simulink model "autosar_tpc_throttle_sensor2"  (R2022a)
settings: Solver=FixedStepDiscrete  StartTime=0.0  StopTime=10.0  FixedStep=0.005  RelTol=1e-3
model workspace (MATLAB code in the model file + MAT data in the model file):
  TPSPercent_LkupTbl = Simulink.LookupTable
  TPSPercent_LkupTbl.Table.DataType = 'single'
  TPSPercent_LkupTbl.Table.Min = []
  TPSPercent_LkupTbl.Table.Max = []
  TPSPercent_LkupTbl.Table.Unit = ''
  TPSPercent_LkupTbl.Table.FieldName = 'Table'
  TPSPercent_LkupTbl.Table.Description = ''
  TPSPercent_LkupTbl.Table.Value = [0 10 20 30 40 50 60 70 80 90 100]
  TPSPercent_LkupTbl.BreakpointsSpecification = 'Explicit values'
  TPSPercent_LkupTbl.SupportTunableSize = false
  TPSPercent_LkupTbl.Breakpoints.DataType = 'single'
  TPSPercent_LkupTbl.Breakpoints.Min = []
  TPSPercent_LkupTbl.Breakpoints.Max = []
  TPSPercent_LkupTbl.Breakpoints.Unit = ''
  TPSPercent_LkupTbl.Breakpoints.FieldName = 'BP1'
  TPSPercent_LkupTbl.Breakpoints.Description = ''
  TPSPercent_LkupTbl.Breakpoints.Value = single(linspace(170, 966, 11))
  TPSPercent_LkupTbl.Breakpoints.TunableSizeName = 'N1'
  TPSPercent_LkupTbl.CoderInfo.StorageClass = 'Auto'
  TPSPercent_LkupTbl.StructTypeInfo.Name = 'MyStruct'
  TPSPercent_LkupTbl.StructTypeInfo.DataScope = 'Auto'
  TPSPercent_LkupTbl.StructTypeInfo.HeaderFileName = ''
  TPSSecondaryPercent_LkupTbl = Simulink.LookupTable
  TPSSecondaryPercent_LkupTbl.Table = Simulink.lookuptable.Table
  TPSSecondaryPercent_LkupTbl.Table.Value = [100 90 80 70 60 50 40 30 20 10 0]
  TPSSecondaryPercent_LkupTbl.Table.Dimensions = [1 11]
  TPSSecondaryPercent_LkupTbl.Table.DataType = 'single'
  TPSSecondaryPercent_LkupTbl.Table.FieldName = 'Table'
  TPSSecondaryPercent_LkupTbl.Breakpoints = Simulink.lookuptable.Breakpoint
  TPSSecondaryPercent_LkupTbl.Breakpoints.Value = [170 249.600006104 329.200012207 408.799987793 488.399993896 568 647.599975586 727.200012207 806.799987793 886.400024414 966]
  TPSSecondaryPercent_LkupTbl.Breakpoints.TunableSizeName = 'N1'
  TPSSecondaryPercent_LkupTbl.Breakpoints.Dimensions = [1 11]
  TPSSecondaryPercent_LkupTbl.Breakpoints.DataType = 'single'
  TPSSecondaryPercent_LkupTbl.Breakpoints.FieldName = 'BP1'
  TPSSecondaryPercent_LkupTbl.SupportTunableSize = 0
  TPSSecondaryPercent_LkupTbl.StructTypeInfo = Simulink.lookuptable.StructTypeInfo
  TPSSecondaryPercent_LkupTbl.StructTypeInfo.Name = 'MyStruct'
  TPSSecondaryPercent_LkupTbl.StructTypeInfo.DataScope = 'Auto'
  TPSSecondaryPercent_LkupTbl.StructTypeInfo.HeaderFileName = 'Rte_Type.h'
undefined symbols (not defined in the file or in its folder): Dem_EventStatusType, TPSPercentBkpt, TPSPercentTbl
libraries: autosarlibdem x2, autosarlibnvm x1
settings Model: Creator=The MathWorks, Inc.  LastModifiedBy=tsen
settings SolverCC: AlgebraicLoopSolver=TrustRegion
settings DataIOCC: ReturnWorkspaceOutputs=off
settings OptimizationCC: DefaultParameterBehavior=Inlined  PassReuseOutputArgsAs=Individual arguments  ZeroExternalMemoryAtStartup=off  ZeroInternalMemoryAtStartup=off  EfficientTunableParamExpr=on
settings DebuggingCC: ParameterTunabilityLossMsg=error  UnconnectedInputMsg=warning  UnconnectedOutputMsg=warning  UnconnectedLineMsg=warning  SFMachineParentedDataDiag=warning  ArithmeticOperatorsInVariantConditions=warning
settings SFSimCC: SimUseLocalCustomCode=off  MATLABDynamicMemAlloc=off
settings RTWCC: Description=AUTOSAR  SystemTargetFile=autosar.tlc  GenCodeOnly=on  TemplateMakefile=ert_default_tmf  GenerateReport=on  RTWVerbose=off  RTWUseLocalCustomCode=off  IncludeHyperlinkInReport=on  LaunchReport=on  GenerateTraceInfo=on  GenerateTraceReport=on  GenerateTraceReportSl=on  GenerateTraceReportSf=on  GenerateTraceReportEml=on
settings CodeAppCC: ForceParamTrailComments=on  IgnoreCustomStorageClasses=off  OperatorAnnotations=on  SimulinkDataObjDesc=on  SFDataObjDesc=on  InsertBlockDesc=on
settings STFCustomTargetCC: TargetLangStandard=C99 (ISO)  MultiwordLength=256  ParMdlRefBuildCompliant=on  CompOptLevelCompliant=on  IncludeMdlTerminateFcn=off  CombineOutputUpdateFcns=on  SuppressErrorStatus=on  ERTCustomFileBanners=on  SupportNonFinite=off  SupportComplex=off  SupportContinuousTime=off  SupportNonInlinedSFcns=off  RemoveResetFunc=on  MATLABClassNameForMDSCustomization=Simulink.SoftwareTarget.ERTCustomization  CPPClassGenCompliant=on  AutosarCompliant=on  GRTInterface=off  UseToolchainInfoCompliant=on  LookupTableObjectStructAxisOrder=2,1,3,4,...  LUTObjectStructOrderEvenSpacing=Size,Table,Breakpoints  SystemTargetFile=autosar.tlc
settings ERTTargetCC: TargetLangStandard=C99 (ISO)  ConcurrentExecutionCompliant=off  IncludeMdlTerminateFcn=off  SuppressErrorStatus=on  SupportNonFinite=off  SupportComplex=off  ModelStepFunctionPrototypeControlCompliant=off  AutosarCompliant=on  LookupTableObjectStructAxisOrder=2,1,3,4,...  LUTObjectStructOrderEvenSpacing=Size,Table,Breakpoints  InlinedParameterPlacement=NonHierarchical  ERTCustomFileTemplate=example_file_process.tlc

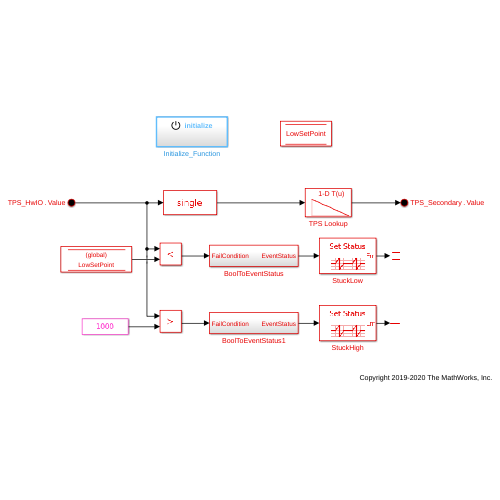
[thumbnail: Simulink's stored preview of the top-level diagram]
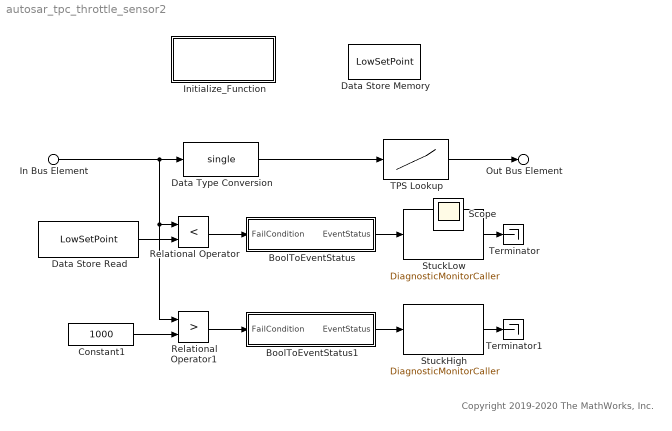
== system autosar_tpc_throttle_sensor2 ==
  note: Copyright 2019-2020 The MathWorks, Inc.
  In Bus Element : Inport  PortName=TPS_HwIO  Element=Value
  BoolToEventStatus : Subsystem
  BoolToEventStatus1 : Subsystem
  Constant1 : Constant  Value=1000
  Data Store Memory : DataStoreMemory  DataStoreName=LowSetPoint  InitialValue=50  ShowAdditionalParam=off
  Data Store Read : DataStoreRead  DataStoreName=LowSetPoint  IndexOptions=Index vector (dialog)  Indices=1  OutputSizes=1
  Data Type Conversion : DataTypeConversion  OutDataTypeStr=single  SaturateOnIntegerOverflow=off  RndMeth=Floor
  Initialize_Function : Subsystem  TreatAsAtomicUnit=on
  Relational Operator : RelationalOperator  Operator=<  OutDataTypeStr=boolean  InputSameDT=off
  Relational Operator1 : RelationalOperator  Operator=>  OutDataTypeStr=boolean  InputSameDT=off
  StuckHigh : autosarlibdem/DiagnosticMonitorCaller  PortName=S2StuckHigh  Operation=SetEventStatus  Datatype=Enum: Dem_EventStatusType  st=-1  ServiceImpl=autosar.bsw.DemDiagnosticMonitor
      settings: SourceProductBaseCode=AS
  StuckLow : autosarlibdem/DiagnosticMonitorCaller  PortName=S2StuckLow  Operation=SetEventStatus  Datatype=Enum: Dem_EventStatusType  st=-1  ServiceImpl=autosar.bsw.DemDiagnosticMonitor
      settings: SourceProductBaseCode=AS
  TPS Lookup : Lookup_n-D  NumberOfTableDimensions=1  DataSpecification=Lookup table object  LookupTableObject=TPSSecondaryPercent_LkupTbl  BreakpointsForDimension1=TPSPercentBkpt  BreakpointsForDimension1DataTypeStr=single  IndexSearchMethod=Linear search  Table=TPSPercentTbl  TableDataTypeStr=single  ExtrapMethod=Clip  InternalRulePriority=Speed  OutDataTypeStr=single  RndMeth=Simplest
  Terminator : Terminator
  Terminator1 : Terminator
  Out Bus Element : Outport  VectorParamsAs1DForOutWhenUnconnected=off  PortName=TPS_Secondary  Element=Value
  Scope : Scope
  wires:
  TPS Lookup/1 -> Out Bus Element/1
  Data Type Conversion/1 -> TPS Lookup/1
  StuckHigh/1 -> Terminator1/1
  Relational Operator/1 -> BoolToEventStatus/1(FailCondition)
  StuckLow/1 -> Terminator/1
  In Bus Element/1 -> Relational Operator1/1, Relational Operator/1, Data Type Conversion/1
  Constant1/1 -> Relational Operator1/2
  Relational Operator1/1 -> BoolToEventStatus1/1(FailCondition)
  BoolToEventStatus/1(EventStatus) -> StuckLow/1
  Data Store Read/1 -> Relational Operator/2
  BoolToEventStatus1/1(EventStatus) -> StuckHigh/1

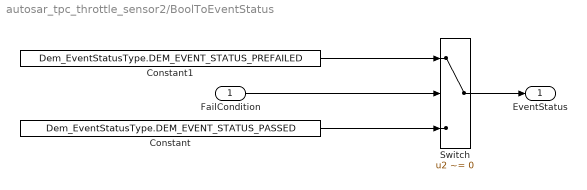
== system autosar_tpc_throttle_sensor2/BoolToEventStatus ==
  FailCondition : Inport
  Constant : Constant  Value=Dem_EventStatusType.DEM_EVENT_STATUS_PASSED
  Constant1 : Constant  Value=Dem_EventStatusType.DEM_EVENT_STATUS_PREFAILED
  Switch : Switch  Criteria=u2 ~= 0  SaturateOnIntegerOverflow=off  InputSameDT=off
  EventStatus : Outport  VectorParamsAs1DForOutWhenUnconnected=off
  wires:
  FailCondition/1 -> Switch/2
  Constant/1 -> Switch/3
  Constant1/1 -> Switch/1
  Switch/1 -> EventStatus/1

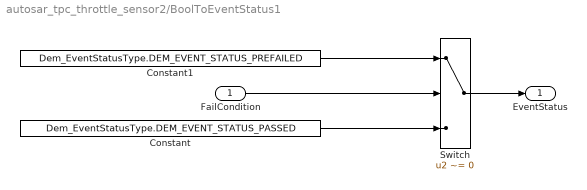
== system autosar_tpc_throttle_sensor2/BoolToEventStatus1 ==
  FailCondition : Inport
  Constant : Constant  Value=Dem_EventStatusType.DEM_EVENT_STATUS_PASSED
  Constant1 : Constant  Value=Dem_EventStatusType.DEM_EVENT_STATUS_PREFAILED
  Switch : Switch  Criteria=u2 ~= 0  SaturateOnIntegerOverflow=off  InputSameDT=off
  EventStatus : Outport  VectorParamsAs1DForOutWhenUnconnected=off
  wires:
  Switch/1 -> EventStatus/1
  Constant1/1 -> Switch/1
  Constant/1 -> Switch/3
  FailCondition/1 -> Switch/2

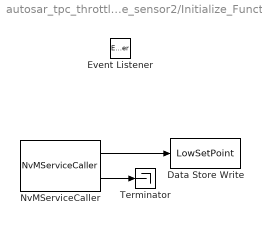
== system autosar_tpc_throttle_sensor2/Initialize_Function ==
  Data Store Write : DataStoreWrite  DataStoreName=LowSetPoint  IndexOptions=Index vector (dialog)  Indices=1  OutputSizes=1
  Event Listener : EventListener  DisableCoverage=on  EventName=reset
  NvMServiceCaller : autosarlibnvm/NvMServiceCaller  PortName=S2LowSetPoint  Operation=ReadBlock  ArgumentSpecification=uint8(1)  st=-1  ServiceImpl=autosar.bsw.NvMService
      settings: SourceProductBaseCode=AS
  Terminator : Terminator
  wires:
  NvMServiceCaller/2 -> Terminator/1
  NvMServiceCaller/1 -> Data Store Write/1
